simulink model "TransparencySimulator"  (R2020a)
settings: Solver=VariableStepAuto  StartTime=0  StopTime=20  FixedStep=0.001  RelTol=1e-3
values from neighbouring files (symbols this model uses):
  A = [0 0 0 1 0 0;      0 0 0 0 1 0;      0 0 0 0 0 1;      -Ka/Jh Ka/Jh 0 0 0 0;     Ka/Je -(Ks + Ka)/Je Ks/Je 0 0 0;      0 Ks/Ja -Ks/Ja 0 0 -Beq/Ja]    [SimulationParam.m]    (also in SimulationParameters.m; abc_ws.mat = [0 0 0 1567.93947765 0 0 0 0 -1685.45584092 221.276595745 0 ; kalmanSS.m = [0 0 0 1 0 0;      0 0 0 0 1 0;      0 0 0 0 0 1;      -Ka/J; kalmanSSHumInput.m = [zeros(1,state_dim);      0 0 0 1 0;      0 0 0 0 1;      Ka)
  A_kf = [0 0 0 0 Ka 0;      0 0 0 0 0 0;      0 0 0 0 1 0;      0 0 0 0 0 1;      0 Ka/Je -(Ks + Ka)/Je Ks/Je 0 0;      0 0 Ks/Ja -Ks/Ja 0 -Beq/Ja]    [SimulationParam.m]    (also in SimulationParameters.m)
  B = [zeros(3,control_dim); 1/Jh 0 0; 0 -1/Je 0; 0 0 N*KI/Ja]    [SimulationParam.m]    (also in SimulationParameters.m; abc_ws.mat = [1 0 0 0 0 0 0 0 -1.12996503145 0 0 0 ... (15 elements, 5x3); kalmanSS.m; kalmanSSHumInput.m = [1 0 0; zeros(2,control_dim); 0 -1/Je 0; 0 0 N*KI/Ja])
  B_kf = [-Ka 0 0; 1 0 0; zeros(2,kf_ctrl_dim); 0 -1/Je 0; 0 0 N*KI/Ja]    [SimulationParam.m]    (also in SimulationParameters.m)
  C = [zeros(sensor_dim,state_dim)]    [SimulationParam.m]    (also in SimulationParameters.m; abc_ws.mat = [-1387.6 0 0 0 0 0 1387.6 0 1 0 0 0 ... (30 elements, 6x5)]; kalmanSS.m; kalmanSSHumInput.m)
  C_kf = [zeros(kf_snr_dim,kf_ste_dim)]    [SimulationParam.m]    (also in SimulationParameters.m)
  CURRENT_MAX = pi    (= 3.14159265359)    [SimulationParam.m]    (also in SimulationParameters.m; abc_ws.mat = 3.14)
  D = zeros(sensor_dim, control_dim)    [SimulationParam.m]    (also in SimulationParameters.m; abc_ws.mat = [0 1 0 0 0 0 0 0 0 0 0 0 ... (18 elements, 6x3)]; kalmanSS.m; kalmanSSHumInput.m = zeros(sensor_dim, control_dim); D(2,1) = 1)
  D_kf = zeros(kf_snr_dim, kf_ctrl_dim); D_kf(2,1) = 1    [SimulationParam.m]    (also in SimulationParameters.m)
  damping_d = 0.001    [SimulationParam.m]    (also in SimulationParameters.m; abc_ws.mat = 0.770835010154; kalmanSSHumInput.m = 0.9)
  dt = 0.001    [SimulationParam.m]    (also in SimulationParameters.m; kalmanSS.m; kalmanSSHumInput.m)
  epos_Ki = 1.190    (= 1.19)    [SimulationParam.m]    (also in SimulationParameters.m; abc_ws.mat; kalmanSSHumInput.m)
  epos_Kp = 11.900    (= 11.9)    [SimulationParam.m]    (also in SimulationParameters.m; abc_ws.mat; kalmanSSHumInput.m)
  Fk = eye(kf_ste_dim) + A_kf*dt + (A_kf*dt)^2/prod(1:2) + (A_kf*dt)^3/prod(1:3) + (A_kf*dt)^4/prod(1:4)    [SimulationParam.m]    (also in SimulationParameters.m; kalmanSS.m = eye(state_dim) + A*dt + (A*dt)^2/prod(1:2) + (A*dt)^3/prod(1; kalmanSSHumInput.m = eye(state_dim) + A*dt + (A*dt)^2/prod(1:2) + (A*dt)^3/prod(1)
  Gk = dt*(eye(kf_ste_dim) + A_kf*dt/prod(1:2) + (A_kf*dt)^2/prod(1:3) + (A_kf*dt)^3/prod(1:4) +         (A_kf*dt)^4/prod(1:5))*B_kf    [SimulationParam.m]    (also in SimulationParameters.m; kalmanSS.m = dt*(eye(state_dim) + A*dt/prod(1:2) + (A*dt)^2/prod(1:3) + (; kalmanSSHumInput.m = dt*(eye(state_dim) + A*dt/prod(1:2) + (A*dt)^2/prod(1:3) + ()
  Ja = 0.47    [SimulationParam.m]    (also in SimulationParameters.m; abc_ws.mat; kalmanSS.m; kalmanSSHumInput.m)
  Je = W*Le^2    (= 0.88498313856)    [SimulationParam.m]    (also in SimulationParameters.m; abc_ws.mat; kalmanSS.m; kalmanSSHumInput.m)
  Jh = 0.0437    [SimulationParam.m]    (also in SimulationParameters.m; abc_ws.mat; kalmanSS.m; kalmanSSHumInput.m)
  k_bar = 1 - stiffness_d/Ks    (= 0.993269230769)    [SimulationParam.m]    (also in SimulationParameters.m)
  kf_ste_dim = 6    [SimulationParam.m]    (also in SimulationParameters.m)
  KI = 0.0603    [SimulationParam.m]    (also in SimulationParameters.m; abc_ws.mat; kalmanSS.m; kalmanSSHumInput.m)
  Ks = 104    [SimulationParam.m]    (also in SimulationParameters.m; abc_ws.mat; kalmanSS.m; kalmanSSHumInput.m)
  Le = 0.432    [SimulationParam.m]    (also in SimulationParameters.m; abc_ws.mat; kalmanSS.m; kalmanSSHumInput.m)
  N = 150    [SimulationParam.m]    (also in SimulationParameters.m; abc_ws.mat; kalmanSS.m; kalmanSSHumInput.m)
  p_e_idx = 3    [SimulationParam.m]    (also in SimulationParameters.m)
  p_m_idx = 4    [SimulationParam.m]    (also in SimulationParameters.m)
  Rk = eye(kf_snr_dim)    [SimulationParam.m]    (also in SimulationParameters.m; kalmanSSnoHum.mat = [9.41238823041e-06 0 0 0 0 5.4756e-06 0 0 0 0 2.3530970576e-)
  stiffness_d = 0.7    [SimulationParam.m]    (also in SimulationParameters.m; abc_ws.mat = 14.0803237251; kalmanSSHumInput.m = 3.874)
  stiffness_lower = damping_d*(epos_Ki/epos_Kp - damping_d/(Ja*k_bar) - epos_Kp/Ja)    (= -0.0252212910136)    [SimulationParam.m]    (also in SimulationParameters.m; abc_ws.mat = -20.9019922533; kalmanSSHumInput.m = -24.4873189611)
  Threaded_Ts = 0.001    [SimulationParam.m]    (also in SimulationParameters.m; abc_ws.mat)
  v_e_idx = 5    [SimulationParam.m]    (also in SimulationParameters.m)
  v_h_idx = 2    [SimulationParam.m]    (also in SimulationParameters.m)
  v_m_idx = 6    [SimulationParam.m]    (also in SimulationParameters.m)
  We = W*g    (= 46.5037717323)    [SimulationParam.m]    (also in SimulationParameters.m; abc_ws.mat; kalmanSS.m; kalmanSSHumInput.m)
undefined symbols (not defined in the file or in its folder): DiscIntNeverNeededParam, Discrete, Time
libraries: simulink x15, simulink_extras x6, dspstat3 x3, ctrlSharedLib x1
(part 2 of 2)

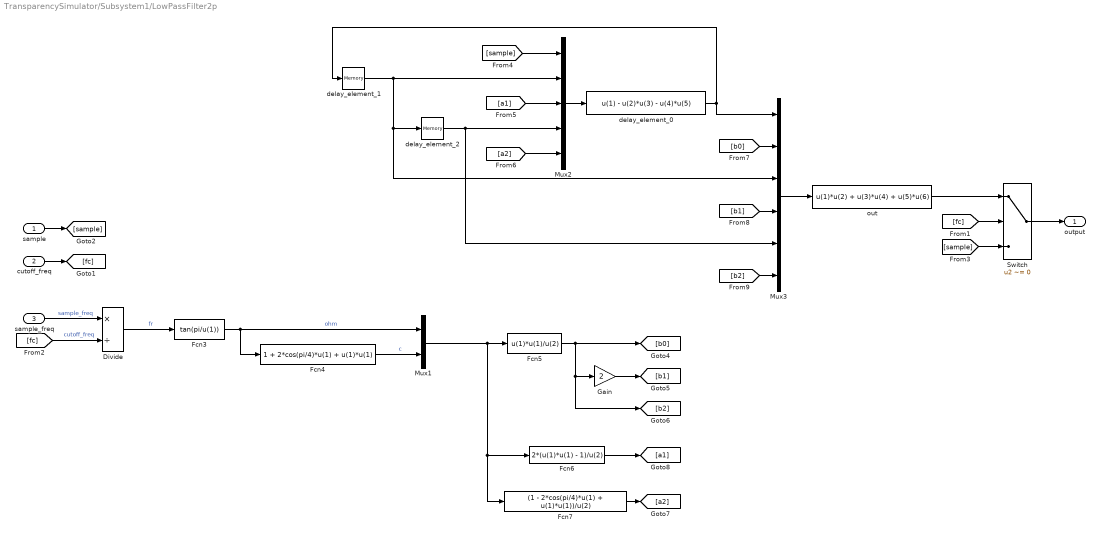
== system TransparencySimulator/Subsystem1/LowPassFilter2p ==
  sample : Inport
  cutoff_freq : Inport  Port=2
  sample_freq : Inport  Port=3
  Divide : Product  Inputs=*/
  Fcn3 : Fcn  Expr=tan(pi/u(1))
  Fcn4 : Fcn  Expr=1 + 2*cos(pi/4)*u(1) + u(1)*u(1)
  Fcn5 : Fcn  Expr=u(1)*u(1)/u(2)
  Fcn6 : Fcn  Expr=2*(u(1)*u(1) - 1)/u(2)
  Fcn7 : Fcn  Expr=(1 - 2*cos(pi/4)*u(1) + u(1)*u(1))/u(2)
  Gain : Gain  Gain=2
  Mux1 : Mux  Inputs=2
  Mux2 : Mux  Inputs=5
  Mux3 : Mux  Inputs=6
  Switch : Switch  Criteria=u2 ~= 0
  delay_element_0 : Fcn  Expr=u(1) - u(2)*u(3) - u(4)*u(5)
  delay_element_1 : Memory  InheritSampleTime=on
  delay_element_2 : Memory  InheritSampleTime=on
  out : Fcn  Expr=u(1)*u(2) + u(3)*u(4) + u(5)*u(6)
  output : Outport
  wires:
  Mux3/1 -> out/1
  [b2] -> Mux3/6
  [b1] -> Mux3/4
  [b0] -> Mux3/2
  delay_element_0/1 -> Mux3/1, delay_element_1/1
  out/1 -> Switch/1
  [a2] -> Mux2/5
  delay_element_2/1 -> Mux3/5, Mux2/4
  [a1] -> Mux2/3
  Mux2/1 -> delay_element_0/1
  [sample] -> Mux2/1
  delay_element_1/1 -> Mux2/2, Mux3/3, delay_element_2/1
  [sample] -> Switch/3
  sample/1 -> [sample]
  Fcn7/1 -> [a2]
  Fcn6/1 -> [a1]
  Gain/1 -> [b1]
  Fcn5/1 -> Gain/1, [b2], [b0]
  Fcn4/1 -> Mux1/2  "c"
  Fcn3/1 -> Fcn4/1, Mux1/1  "ohm"
  Mux1/1 -> Fcn5/1, Fcn6/1, Fcn7/1
  Divide/1 -> Fcn3/1  "fr"
  [fc] -> Divide/2  "cutoff_freq"
  sample_freq/1 -> Divide/1  "sample_freq"
  [fc] -> Switch/2
  cutoff_freq/1 -> [fc]
  Switch/1 -> output/1

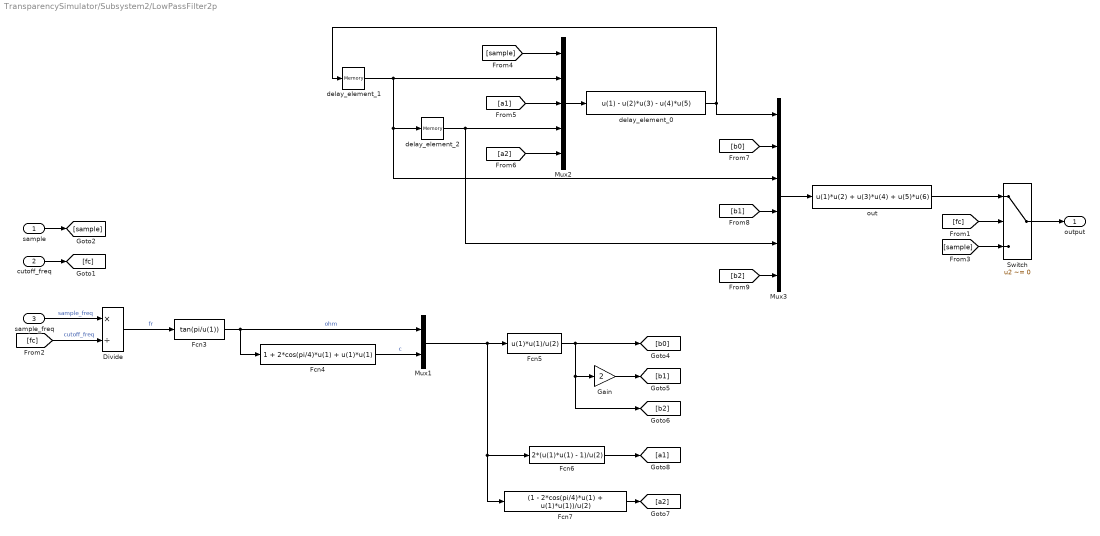
== system TransparencySimulator/Subsystem2/LowPassFilter2p ==
  sample : Inport
  cutoff_freq : Inport  Port=2
  sample_freq : Inport  Port=3
  Divide : Product  Inputs=*/
  Fcn3 : Fcn  Expr=tan(pi/u(1))
  Fcn4 : Fcn  Expr=1 + 2*cos(pi/4)*u(1) + u(1)*u(1)
  Fcn5 : Fcn  Expr=u(1)*u(1)/u(2)
  Fcn6 : Fcn  Expr=2*(u(1)*u(1) - 1)/u(2)
  Fcn7 : Fcn  Expr=(1 - 2*cos(pi/4)*u(1) + u(1)*u(1))/u(2)
  Gain : Gain  Gain=2
  Mux1 : Mux  Inputs=2
  Mux2 : Mux  Inputs=5
  Mux3 : Mux  Inputs=6
  Switch : Switch  Criteria=u2 ~= 0
  delay_element_0 : Fcn  Expr=u(1) - u(2)*u(3) - u(4)*u(5)
  delay_element_1 : Memory  InheritSampleTime=on
  delay_element_2 : Memory  InheritSampleTime=on
  out : Fcn  Expr=u(1)*u(2) + u(3)*u(4) + u(5)*u(6)
  output : Outport
  wires:
  Mux3/1 -> out/1
  [b2] -> Mux3/6
  [b1] -> Mux3/4
  [b0] -> Mux3/2
  delay_element_0/1 -> Mux3/1, delay_element_1/1
  out/1 -> Switch/1
  [a2] -> Mux2/5
  delay_element_2/1 -> Mux3/5, Mux2/4
  [a1] -> Mux2/3
  Mux2/1 -> delay_element_0/1
  [sample] -> Mux2/1
  delay_element_1/1 -> Mux2/2, Mux3/3, delay_element_2/1
  [sample] -> Switch/3
  sample/1 -> [sample]
  Fcn7/1 -> [a2]
  Fcn6/1 -> [a1]
  Gain/1 -> [b1]
  Fcn5/1 -> Gain/1, [b2], [b0]
  Fcn4/1 -> Mux1/2  "c"
  Fcn3/1 -> Fcn4/1, Mux1/1  "ohm"
  Mux1/1 -> Fcn5/1, Fcn6/1, Fcn7/1
  Divide/1 -> Fcn3/1  "fr"
  [fc] -> Divide/2  "cutoff_freq"
  sample_freq/1 -> Divide/1  "sample_freq"
  [fc] -> Switch/2
  cutoff_freq/1 -> [fc]
  Switch/1 -> output/1

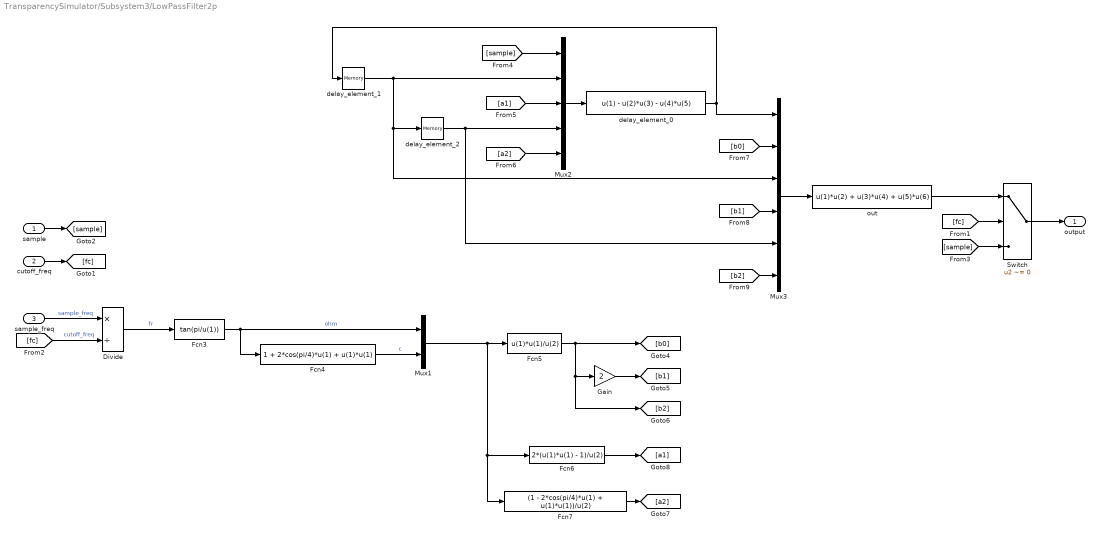
== system TransparencySimulator/Subsystem3/LowPassFilter2p ==
  sample : Inport
  cutoff_freq : Inport  Port=2
  sample_freq : Inport  Port=3
  Divide : Product  Inputs=*/
  Fcn3 : Fcn  Expr=tan(pi/u(1))
  Fcn4 : Fcn  Expr=1 + 2*cos(pi/4)*u(1) + u(1)*u(1)
  Fcn5 : Fcn  Expr=u(1)*u(1)/u(2)
  Fcn6 : Fcn  Expr=2*(u(1)*u(1) - 1)/u(2)
  Fcn7 : Fcn  Expr=(1 - 2*cos(pi/4)*u(1) + u(1)*u(1))/u(2)
  Gain : Gain  Gain=2
  Mux1 : Mux  Inputs=2
  Mux2 : Mux  Inputs=5
  Mux3 : Mux  Inputs=6
  Switch : Switch  Criteria=u2 ~= 0
  delay_element_0 : Fcn  Expr=u(1) - u(2)*u(3) - u(4)*u(5)
  delay_element_1 : Memory  InheritSampleTime=on
  delay_element_2 : Memory  InheritSampleTime=on
  out : Fcn  Expr=u(1)*u(2) + u(3)*u(4) + u(5)*u(6)
  output : Outport
  wires:
  Mux3/1 -> out/1
  [b2] -> Mux3/6
  [b1] -> Mux3/4
  [b0] -> Mux3/2
  delay_element_0/1 -> Mux3/1, delay_element_1/1
  out/1 -> Switch/1
  [a2] -> Mux2/5
  delay_element_2/1 -> Mux3/5, Mux2/4
  [a1] -> Mux2/3
  Mux2/1 -> delay_element_0/1
  [sample] -> Mux2/1
  delay_element_1/1 -> Mux2/2, Mux3/3, delay_element_2/1
  [sample] -> Switch/3
  sample/1 -> [sample]
  Fcn7/1 -> [a2]
  Fcn6/1 -> [a1]
  Gain/1 -> [b1]
  Fcn5/1 -> Gain/1, [b2], [b0]
  Fcn4/1 -> Mux1/2  "c"
  Fcn3/1 -> Fcn4/1, Mux1/1  "ohm"
  Mux1/1 -> Fcn5/1, Fcn6/1, Fcn7/1
  Divide/1 -> Fcn3/1  "fr"
  [fc] -> Divide/2  "cutoff_freq"
  sample_freq/1 -> Divide/1  "sample_freq"
  [fc] -> Switch/2
  cutoff_freq/1 -> [fc]
  Switch/1 -> output/1

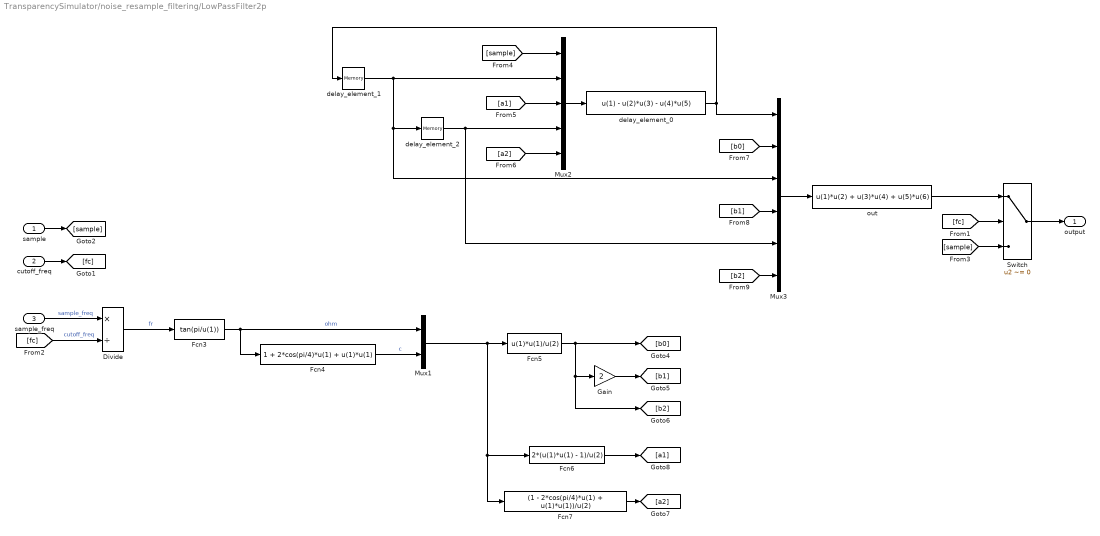
== system TransparencySimulator/noise_resample_filtering/LowPassFilter2p ==
  sample : Inport
  cutoff_freq : Inport  Port=2
  sample_freq : Inport  Port=3
  Divide : Product  Inputs=*/
  Fcn3 : Fcn  Expr=tan(pi/u(1))
  Fcn4 : Fcn  Expr=1 + 2*cos(pi/4)*u(1) + u(1)*u(1)
  Fcn5 : Fcn  Expr=u(1)*u(1)/u(2)
  Fcn6 : Fcn  Expr=2*(u(1)*u(1) - 1)/u(2)
  Fcn7 : Fcn  Expr=(1 - 2*cos(pi/4)*u(1) + u(1)*u(1))/u(2)
  Gain : Gain  Gain=2
  Mux1 : Mux  Inputs=2
  Mux2 : Mux  Inputs=5
  Mux3 : Mux  Inputs=6
  Switch : Switch  Criteria=u2 ~= 0
  delay_element_0 : Fcn  Expr=u(1) - u(2)*u(3) - u(4)*u(5)
  delay_element_1 : Memory  InheritSampleTime=on
  delay_element_2 : Memory  InheritSampleTime=on
  out : Fcn  Expr=u(1)*u(2) + u(3)*u(4) + u(5)*u(6)
  output : Outport
  wires:
  Switch/1 -> output/1
  cutoff_freq/1 -> [fc]
  [fc] -> Switch/2
  sample_freq/1 -> Divide/1  "sample_freq"
  [fc] -> Divide/2  "cutoff_freq"
  Divide/1 -> Fcn3/1  "fr"
  Mux1/1 -> Fcn7/1, Fcn6/1, Fcn5/1
  Fcn3/1 -> Mux1/1, Fcn4/1  "ohm"
  Fcn4/1 -> Mux1/2  "c"
  Fcn5/1 -> [b0], [b2], Gain/1
  Gain/1 -> [b1]
  Fcn6/1 -> [a1]
  Fcn7/1 -> [a2]
  sample/1 -> [sample]
  [sample] -> Switch/3
  delay_element_1/1 -> delay_element_2/1, Mux3/3, Mux2/2
  [sample] -> Mux2/1
  Mux2/1 -> delay_element_0/1
  [a1] -> Mux2/3
  delay_element_2/1 -> Mux2/4, Mux3/5
  [a2] -> Mux2/5
  out/1 -> Switch/1
  delay_element_0/1 -> delay_element_1/1, Mux3/1
  [b0] -> Mux3/2
  [b1] -> Mux3/4
  [b2] -> Mux3/6
  Mux3/1 -> out/1

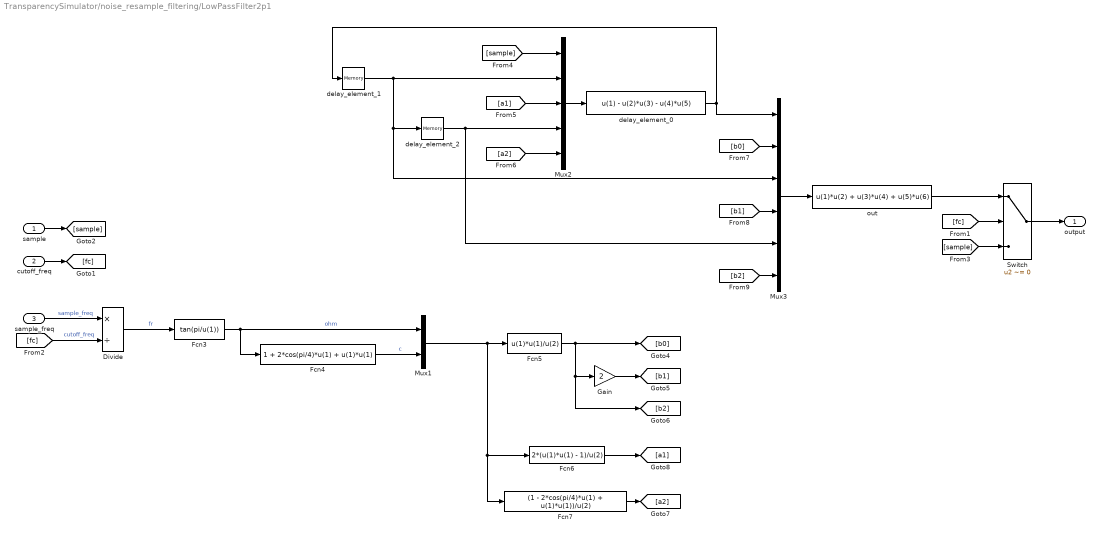
== system TransparencySimulator/noise_resample_filtering/LowPassFilter2p1 ==
  sample : Inport
  cutoff_freq : Inport  Port=2
  sample_freq : Inport  Port=3
  Divide : Product  Inputs=*/
  Fcn3 : Fcn  Expr=tan(pi/u(1))
  Fcn4 : Fcn  Expr=1 + 2*cos(pi/4)*u(1) + u(1)*u(1)
  Fcn5 : Fcn  Expr=u(1)*u(1)/u(2)
  Fcn6 : Fcn  Expr=2*(u(1)*u(1) - 1)/u(2)
  Fcn7 : Fcn  Expr=(1 - 2*cos(pi/4)*u(1) + u(1)*u(1))/u(2)
  Gain : Gain  Gain=2
  Mux1 : Mux  Inputs=2
  Mux2 : Mux  Inputs=5
  Mux3 : Mux  Inputs=6
  Switch : Switch  Criteria=u2 ~= 0
  delay_element_0 : Fcn  Expr=u(1) - u(2)*u(3) - u(4)*u(5)
  delay_element_1 : Memory  InheritSampleTime=on
  delay_element_2 : Memory  InheritSampleTime=on
  out : Fcn  Expr=u(1)*u(2) + u(3)*u(4) + u(5)*u(6)
  output : Outport
  wires:
  Mux3/1 -> out/1
  [b2] -> Mux3/6
  [b1] -> Mux3/4
  [b0] -> Mux3/2
  delay_element_0/1 -> Mux3/1, delay_element_1/1
  out/1 -> Switch/1
  [a2] -> Mux2/5
  delay_element_2/1 -> Mux3/5, Mux2/4
  [a1] -> Mux2/3
  Mux2/1 -> delay_element_0/1
  [sample] -> Mux2/1
  delay_element_1/1 -> Mux2/2, Mux3/3, delay_element_2/1
  [sample] -> Switch/3
  sample/1 -> [sample]
  Fcn7/1 -> [a2]
  Fcn6/1 -> [a1]
  Gain/1 -> [b1]
  Fcn5/1 -> Gain/1, [b2], [b0]
  Fcn4/1 -> Mux1/2  "c"
  Fcn3/1 -> Fcn4/1, Mux1/1  "ohm"
  Mux1/1 -> Fcn5/1, Fcn6/1, Fcn7/1
  Divide/1 -> Fcn3/1  "fr"
  [fc] -> Divide/2  "cutoff_freq"
  sample_freq/1 -> Divide/1  "sample_freq"
  [fc] -> Switch/2
  cutoff_freq/1 -> [fc]
  Switch/1 -> output/1

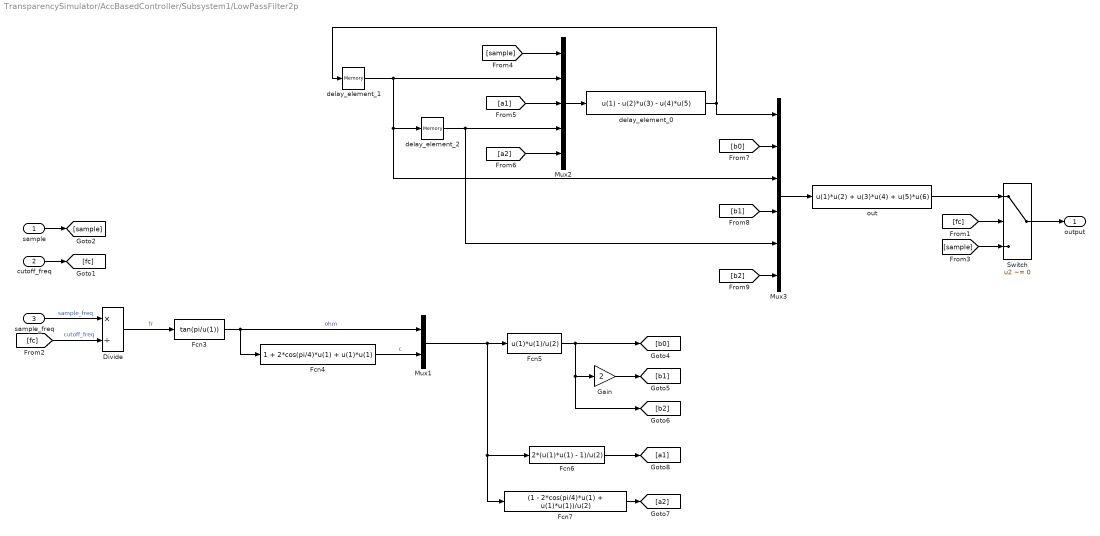
== system TransparencySimulator/AccBasedController/Subsystem1/LowPassFilter2p ==
  sample : Inport
  cutoff_freq : Inport  Port=2
  sample_freq : Inport  Port=3
  Divide : Product  Inputs=*/
  Fcn3 : Fcn  Expr=tan(pi/u(1))
  Fcn4 : Fcn  Expr=1 + 2*cos(pi/4)*u(1) + u(1)*u(1)
  Fcn5 : Fcn  Expr=u(1)*u(1)/u(2)
  Fcn6 : Fcn  Expr=2*(u(1)*u(1) - 1)/u(2)
  Fcn7 : Fcn  Expr=(1 - 2*cos(pi/4)*u(1) + u(1)*u(1))/u(2)
  Gain : Gain  Gain=2
  Mux1 : Mux  Inputs=2
  Mux2 : Mux  Inputs=5
  Mux3 : Mux  Inputs=6
  Switch : Switch  Criteria=u2 ~= 0
  delay_element_0 : Fcn  Expr=u(1) - u(2)*u(3) - u(4)*u(5)
  delay_element_1 : Memory  InheritSampleTime=on
  delay_element_2 : Memory  InheritSampleTime=on
  out : Fcn  Expr=u(1)*u(2) + u(3)*u(4) + u(5)*u(6)
  output : Outport
  wires:
  Switch/1 -> output/1
  cutoff_freq/1 -> [fc]
  [fc] -> Switch/2
  sample_freq/1 -> Divide/1  "sample_freq"
  [fc] -> Divide/2  "cutoff_freq"
  Divide/1 -> Fcn3/1  "fr"
  Mux1/1 -> Fcn7/1, Fcn6/1, Fcn5/1
  Fcn3/1 -> Mux1/1, Fcn4/1  "ohm"
  Fcn4/1 -> Mux1/2  "c"
  Fcn5/1 -> [b0], [b2], Gain/1
  Gain/1 -> [b1]
  Fcn6/1 -> [a1]
  Fcn7/1 -> [a2]
  sample/1 -> [sample]
  [sample] -> Switch/3
  delay_element_1/1 -> delay_element_2/1, Mux3/3, Mux2/2
  [sample] -> Mux2/1
  Mux2/1 -> delay_element_0/1
  [a1] -> Mux2/3
  delay_element_2/1 -> Mux2/4, Mux3/5
  [a2] -> Mux2/5
  out/1 -> Switch/1
  delay_element_0/1 -> delay_element_1/1, Mux3/1
  [b0] -> Mux3/2
  [b1] -> Mux3/4
  [b2] -> Mux3/6
  Mux3/1 -> out/1

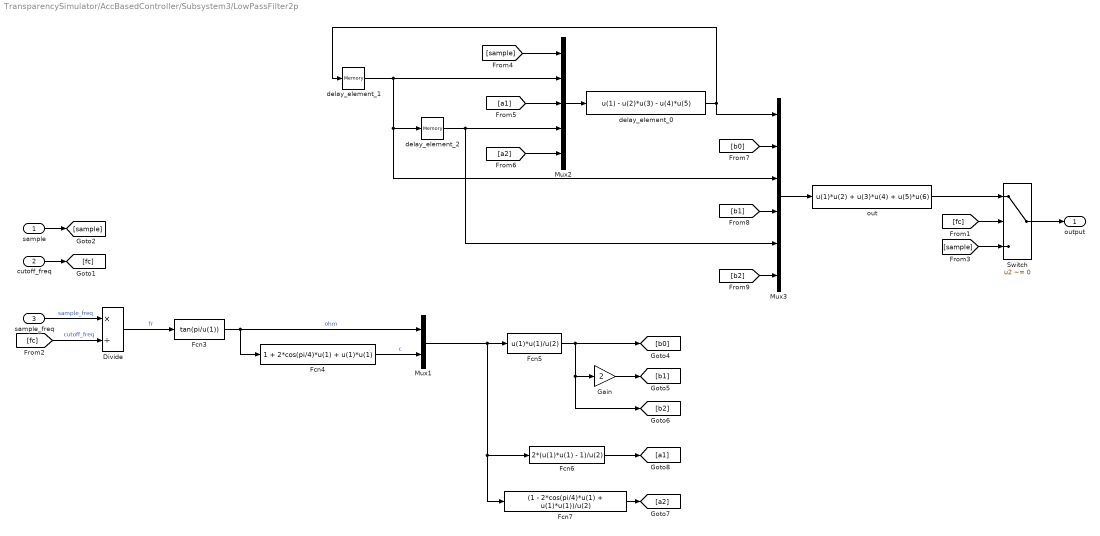
== system TransparencySimulator/AccBasedController/Subsystem3/LowPassFilter2p ==
  sample : Inport
  cutoff_freq : Inport  Port=2
  sample_freq : Inport  Port=3
  Divide : Product  Inputs=*/
  Fcn3 : Fcn  Expr=tan(pi/u(1))
  Fcn4 : Fcn  Expr=1 + 2*cos(pi/4)*u(1) + u(1)*u(1)
  Fcn5 : Fcn  Expr=u(1)*u(1)/u(2)
  Fcn6 : Fcn  Expr=2*(u(1)*u(1) - 1)/u(2)
  Fcn7 : Fcn  Expr=(1 - 2*cos(pi/4)*u(1) + u(1)*u(1))/u(2)
  Gain : Gain  Gain=2
  Mux1 : Mux  Inputs=2
  Mux2 : Mux  Inputs=5
  Mux3 : Mux  Inputs=6
  Switch : Switch  Criteria=u2 ~= 0
  delay_element_0 : Fcn  Expr=u(1) - u(2)*u(3) - u(4)*u(5)
  delay_element_1 : Memory  InheritSampleTime=on
  delay_element_2 : Memory  InheritSampleTime=on
  out : Fcn  Expr=u(1)*u(2) + u(3)*u(4) + u(5)*u(6)
  output : Outport
  wires:
  Mux3/1 -> out/1
  [b2] -> Mux3/6
  [b1] -> Mux3/4
  [b0] -> Mux3/2
  delay_element_0/1 -> Mux3/1, delay_element_1/1
  out/1 -> Switch/1
  [a2] -> Mux2/5
  delay_element_2/1 -> Mux3/5, Mux2/4
  [a1] -> Mux2/3
  Mux2/1 -> delay_element_0/1
  [sample] -> Mux2/1
  delay_element_1/1 -> Mux2/2, Mux3/3, delay_element_2/1
  [sample] -> Switch/3
  sample/1 -> [sample]
  Fcn7/1 -> [a2]
  Fcn6/1 -> [a1]
  Gain/1 -> [b1]
  Fcn5/1 -> Gain/1, [b2], [b0]
  Fcn4/1 -> Mux1/2  "c"
  Fcn3/1 -> Fcn4/1, Mux1/1  "ohm"
  Mux1/1 -> Fcn5/1, Fcn6/1, Fcn7/1
  Divide/1 -> Fcn3/1  "fr"
  [fc] -> Divide/2  "cutoff_freq"
  sample_freq/1 -> Divide/1  "sample_freq"
  [fc] -> Switch/2
  cutoff_freq/1 -> [fc]
  Switch/1 -> output/1
